simulink model "Buck_Converter"  (R2024a)
settings: Solver=FixedStepDiscrete  StartTime=0.0  StopTime=10  FixedStep=1e-5  RelTol=1e-3
InitFcn:
  | Vs = 12;
  | Vref = 5;
  | fs=33e3;
  | L=1e-1;
  | RL=0.015;
  | C=1e-3;
  | RC=0.017;
  | RLoad = 1;
libraries: spsSeriesRLCBranchLib x3, instrumentlib x2, slrealtimeutilitieslib x1, spsCurrentMeasurementLib x1, spsDCVoltageSourceLib x1, spsDiodeLib x1, spsIGBTLib x1, spsPWMGeneratorDCDCLib x1, spsVoltageMeasurementLib x1, spspowerguiLib x1
settings Model: Creator=pvm8318  LastModifiedBy=pvm8318
settings DebuggingCC: UnconnectedInputMsg=warning  UnconnectedOutputMsg=warning  UnconnectedLineMsg=warning
settings ModelReferenceCC: EnableRefExpFcnMdlSchedulingChecks=on
settings RTWCC: GPUComputeCapability=3.5  DLArmComputeVersion=19.05

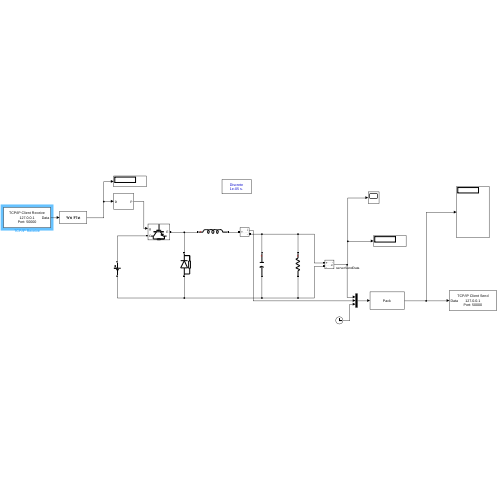
[thumbnail: Simulink's stored preview of the top-level diagram]
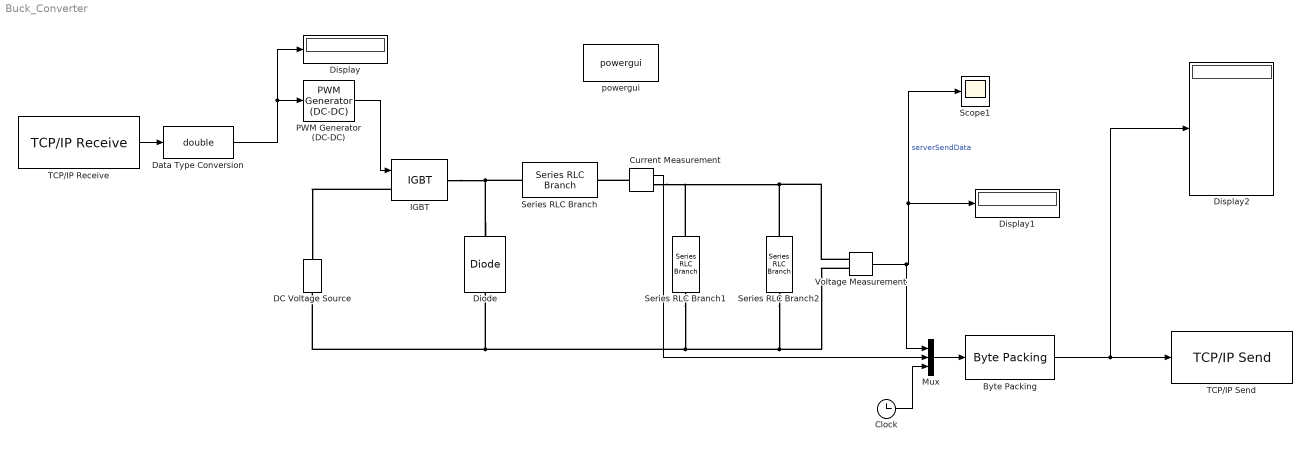
== system Buck_Converter ==
  Byte Packing : slrealtimeutilitieslib/Byte Packing  MaskPackedDataType=double  MaskUnpackedDataTypes={'double'}  MaskAlignment=1
  Clock : Clock
  Current Measurement : spsCurrentMeasurementLib/Current Measurement  PhasorSimulation=off  OutputType=Complex  PSBequivalent=0
  DC Voltage Source : spsDCVoltageSourceLib/DC Voltage Source  Amplitude=Vs  Measurements=None
  Data Type Conversion : DataTypeConversion  OutDataTypeStr=double  SaturateOnIntegerOverflow=off  RndMeth=Floor
  Diode : spsDiodeLib/Diode  Ron=0.001  Lon=0  Vf=0.8  IC=0  UseSnubber=0  Rs=500  Cs=250e-9  Measurements=off
  Display : Display
  Display1 : Display
  Display2 : Display
  IGBT : spsIGBTLib/IGBT  Ron=0.001  Lon=0  Vf=1  Tf=1e-6  Tt=2e-6  IC=0  Rs=1e5  Cs=inf  Measurements=off
  Mux : Mux  Inputs=3
  PWM Generator (DC-DC) : spsPWMGeneratorDCDCLib/PWM Generator (DC-DC)  Fsw=fs  Ts=1e-5
  Scope1 : Scope
  Series RLC Branch : spsSeriesRLCBranchLib/Series RLC Branch  LConnTagsString=__new0  RConnTagsString=__new0  BranchType=L  Resistance=RL  Inductance=L  SetiL0=off  InitialCurrent=0  Capacitance=1e-6  Setx0=off  InitialVoltage=0  Measurements=None
  Series RLC Branch1 : spsSeriesRLCBranchLib/Series RLC Branch  LConnTagsString=__new0  RConnTagsString=__new0  BranchType=C  Resistance=RC  Inductance=1e-3  SetiL0=off  InitialCurrent=0  Capacitance=C  Setx0=off  InitialVoltage=0  Measurements=None
  Series RLC Branch2 : spsSeriesRLCBranchLib/Series RLC Branch  LConnTagsString=__new0  RConnTagsString=__new0  BranchType=R  Resistance=RLoad  Inductance=1e-3  SetiL0=off  InitialCurrent=0  Capacitance=1e-6  Setx0=off  InitialVoltage=0  Measurements=None
  TCP/IP Receive : instrumentlib/TCP//IP Receive  Host=127.0.0.1  Port=50000  DataSize=[ 1, 1 ]  DataType=double  ASCIIFormatting=%f  Terminator=LF  CustomTerminator=10  ByteOrder=big-endian  EnableBlockingMode=on  Timeout=10  SampleTime=1e-4  SimulateUsing=Interpreted execution
  TCP/IP Send : instrumentlib/TCP//IP Send  Host=127.0.0.1  Port=50000  ByteOrder=big-endian  EnableBlockingMode=on  Timeout=10  TransferDelay=on  SimulateUsing=Interpreted execution
  Voltage Measurement : spsVoltageMeasurementLib/Voltage Measurement  PhasorSimulation=off  OutputType=Complex  PSBequivalent=0
  powergui : spspowerguiLib/powergui  Priority=1  SimulationMode=Discrete  SampleTime=1e-5  frequency=60  Iterations=50  frequencyindice=0  Pbase=100e6  ErrMax=1e-4  UnitsV=kV  UnitsW=MW  buscounter=0  FunctionMessages=off  echomessages=off  EnableUseOfTLC=off  CurrentSourceSwitches=off  DisableSnubberDevices=off  DisableRonSwitches=off  DisableVfSwitches=off  DisplayEquations=off  AutomaticDiscreteSolvers=off  SolverType=Tustin/Backward Euler (TBE)  Interpol=off  ExternalGateDelay=off  methode=off  Ts=100  x0status=blocks  SPID=on  SwTol=0  HookPort=off  NonlinearTolerance=1e-4  nMaxIteration=100  ContinueOnMaxIteration=off  RestoreLinks=warning  ResistiveCurrentMeasurement=off  Frange=[0:2:500]  Ylog=off  Xlog=on  ShowGrid=off  save=off  variable=ZData  structure=0  ZoomFFT=off  StartTime=0.0  cycles=1  DisplayStyle=1  fundamental=60  FreqAxis=off  MaxFrequency=1000  frequencyindicesteady=1  RmsSteady=1  display=off
  wires:
  PWM Generator (DC-DC)/1 -> IGBT/1
  Voltage Measurement/1 -> Mux/1, Display1/1, Scope1/1  "serverSendData"
  TCP/IP Receive/1 -> Data Type Conversion/1
  Byte Packing/1 -> TCP/IP Send/1, Display2/1
  Mux/1 -> Byte Packing/1
  Current Measurement/1 -> Mux/2
  Data Type Conversion/1 -> Display/1, PWM Generator (DC-DC)/1
  Clock/1 -> Mux/3
  connections:
  Diode/RConn1 -- Series RLC Branch/LConn1 -- IGBT/RConn1
  Series RLC Branch2/RConn1 -- Series RLC Branch1/RConn1 -- DC Voltage Source/LConn1 -- Diode/LConn1 -- Voltage Measurement/LConn2
  Voltage Measurement/LConn1 -- Current Measurement/RConn1 -- Series RLC Branch1/LConn1 -- Series RLC Branch2/LConn1
  IGBT/LConn1 -- DC Voltage Source/RConn1
  Current Measurement/LConn1 -- Series RLC Branch/RConn1
